simulink model "chap7_6sim"  (Simulink 8.1)
settings: Solver=ode45  StartTime=0.0  StopTime=30  RelTol=1e-5
settings Model: Creator=ljk  LastModifiedBy=liujk  ExtModeTrigMode=oneshot  ExtModeArmWhenConnect=off
settings DataIOCC: LimitDataPoints=off  SignalLoggingName=sigsOut
settings OptimizationCC: BooleanDataType=off  InitFltsAndDblsToZero=on
settings DebuggingCC: SaveWithParameterizedLinksMsg=none  SignalResolutionControl=TryResolveAllWithWarning  SolverPrmCheckMsg=none  MultiTaskDSMMsg=warning  MultiTaskCondExecSysMsg=none  StrictBusMsg=None
settings HardwareCC: TargetUnknown=on
settings RTWCC: IncludeERTFirstTime=on
settings GRTTargetCC: TargetFcnLib=ansi_tfl_tmw.mat

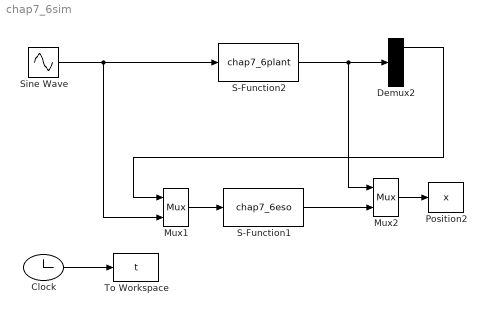
== system chap7_6sim ==
  Clock : Clock
  Demux2 : Demux  Outputs=3
  Mux1 : Mux  Inputs=2
  Mux2 : Mux  Inputs=2
  Position2 : ToWorkspace  VariableName=x  SampleTime=-1
  S-Function1 : S-Function  FunctionName=chap7_6eso  EnableBusSupport=off
  S-Function2 : S-Function  FunctionName=chap7_6plant  EnableBusSupport=off
  Sine Wave : Sin  Amplitude=0.1  SampleTime=0
  To Workspace : ToWorkspace  VariableName=t  SampleTime=-1
  wires:
  Clock/1 -> To Workspace/1
  Sine Wave/1 -> S-Function2/1, Mux1/2
  S-Function2/1 -> Demux2/1, Mux2/1
  Mux1/1 -> S-Function1/1
  Demux2/1 -> Mux1/1
  Mux2/1 -> Position2/1
  S-Function1/1 -> Mux2/2
